simulink model "ThreecellsSolarArray"  (R2016a)
settings: Solver=VariableStepAuto  StartTime=0.0  StopTime=10.0  RelTol=1e-3
libraries: cstblocks x3
settings Model: Creator=f.sanfedino  LastModifiedBy=f.sanfedino

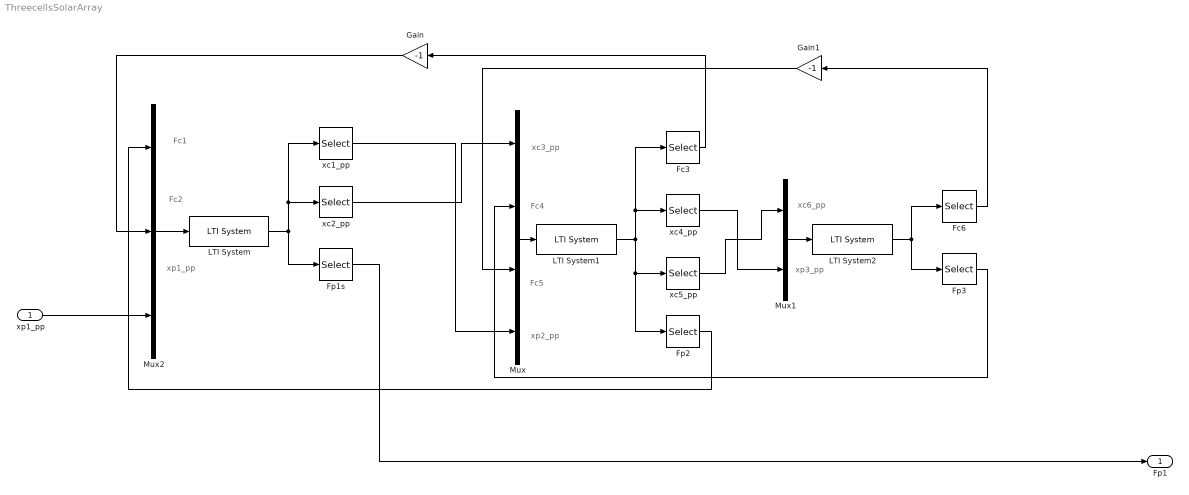
== system ThreecellsSolarArray ==
  note: xp1_pp
  note: Fc2
  note: Fc1
  note: xp3_pp
  note: xc6_pp
  note: xp2_pp
  note: Fc5
  note: Fc4
  note: xc3_pp
  xp1_pp : Inport  PortDimensions=3
  Fc3 : Selector  InputPortWidth=12  IndexOptions=Index vector (dialog)  Indices=[1:3]  OutputSizes=1
  Fc6 : Selector  InputPortWidth=6  IndexOptions=Index vector (dialog)  Indices=[1:3]  OutputSizes=1
  Fp1s : Selector  InputPortWidth=9  IndexOptions=Index vector (dialog)  Indices=[7:9]  OutputSizes=1
  Fp2 : Selector  InputPortWidth=12  IndexOptions=Index vector (dialog)  Indices=[10:12]  OutputSizes=1
  Fp3 : Selector  InputPortWidth=6  IndexOptions=Index vector (dialog)  Indices=[4:6]  OutputSizes=1
  Gain : Gain  Gain=-1
  Gain1 : Gain  Gain=-1
  LTI System : cstblocks/LTI System  sys=M1  IC=[]
  LTI System1 : cstblocks/LTI System  sys=M2_inv  IC=[]
  LTI System2 : cstblocks/LTI System  sys=M3_inv  IC=[]
  Mux : Mux
  Mux1 : Mux  Inputs=2
  Mux2 : Mux  Inputs=3
  xc1_pp : Selector  InputPortWidth=9  IndexOptions=Index vector (dialog)  Indices=[1:3]  OutputSizes=1
  xc2_pp : Selector  InputPortWidth=9  IndexOptions=Index vector (dialog)  Indices=[4:6]  OutputSizes=1
  xc4_pp : Selector  InputPortWidth=12  IndexOptions=Index vector (dialog)  Indices=[4:6]  OutputSizes=1
  xc5_pp : Selector  InputPortWidth=12  IndexOptions=Index vector (dialog)  Indices=[7:9]  OutputSizes=1
  Fp1 : Outport
  wires:
  LTI System/1 -> xc2_pp/1, xc1_pp/1, Fp1s/1
  LTI System1/1 -> xc4_pp/1, Fc3/1, Fp2/1, xc5_pp/1
  LTI System2/1 -> Fp3/1, Fc6/1
  Mux/1 -> LTI System1/1
  xc2_pp/1 -> Mux/1
  xc1_pp/1 -> Mux/4
  Mux1/1 -> LTI System2/1
  xc4_pp/1 -> Mux1/2
  xc5_pp/1 -> Mux1/1
  Fc6/1 -> Gain1/1
  Mux2/1 -> LTI System/1
  xp1_pp/1 -> Mux2/3
  Fc3/1 -> Gain/1
  Fp1s/1 -> Fp1/1
  Gain/1 -> Mux2/2
  Fp2/1 -> Mux2/1
  Fp3/1 -> Mux/2
  Gain1/1 -> Mux/3
